simulink model "Assignment2Problem2_2"  (R2017b)
settings: Solver=VariableStepAuto  StartTime=0.0  StopTime=10.0  RelTol=1e-3
values from neighbouring files (symbols this model uses):
  den = [1 -1.5 -0.9]    [Assignment2Problem2.m]
  num = [2 -3 4]    [Assignment2Problem2.m]
libraries: simulink_extras x1
settings Model: Creator=alexbenasutti  LastModifiedBy=alexbenasutti

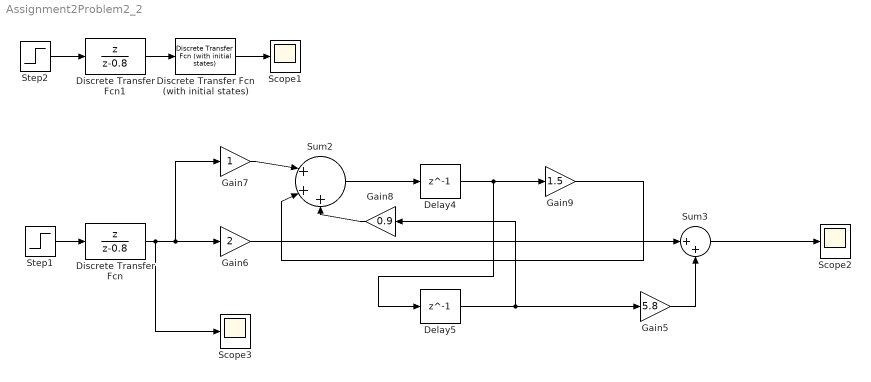
== system Assignment2Problem2_2 ==
  Delay4 : Delay  DelayLength=1  InitialCondition=0
  Delay5 : Delay  DelayLength=1  InitialCondition=0
  Discrete Transfer Fcn : DiscreteTransferFcn  Numerator=[1 0]  Denominator=[1 -0.8]
  Discrete Transfer Fcn (with initial states) : simulink_extras/Additional Discrete/Discrete Transfer Fcn (with initial states)  N=num  D=den  X0=[0 0]  TS=.5
      settings: SourceProductName=Simulink  SourceProductBaseCode=SL
  Discrete Transfer Fcn1 : DiscreteTransferFcn  Numerator=[1 0]  Denominator=[1 -0.8]
  Gain5 : Gain  Gain=5.8
  Gain6 : Gain  Gain=2
  Gain7 : Gain
  Gain8 : Gain  Gain=0.9
  Gain9 : Gain  Gain=1.5
  Scope1 : Scope
  Scope2 : Scope
  Scope3 : Scope
  Step1 : Step  SampleTime=0
  Step2 : Step  SampleTime=0
  Sum2 : Sum  Inputs=|+++
  Sum3 : Sum  Inputs=|++
  wires:
  Step1/1 -> Discrete Transfer Fcn/1
  Discrete Transfer Fcn (with initial states)/1 -> Scope1/1
  Gain5/1 -> Sum3/2
  Delay5/1 -> Gain8/1, Gain5/1
  Discrete Transfer Fcn/1 -> Gain7/1, Gain6/1, Scope3/1
  Gain6/1 -> Sum3/1
  Gain7/1 -> Sum2/1
  Sum2/1 -> Delay4/1
  Delay4/1 -> Gain9/1, Delay5/1
  Gain8/1 -> Sum2/3
  Gain9/1 -> Sum2/2
  Discrete Transfer Fcn1/1 -> Discrete Transfer Fcn (with initial states)/1
  Step2/1 -> Discrete Transfer Fcn1/1
  Sum3/1 -> Scope2/1
